simulink model "BasePendulumSim"  (R2018b)
settings: Solver=VariableStepAuto  StartTime=0.0  StopTime=time(end)  RelTol=1e-3
values from neighbouring files (symbols this model uses):
  B = 0.25    [BasePendulumTest.m]
  g = 9.81    [BasePendulumTest.m]    (also in FeedbackSimOptimization.m; FeedbackSimTest.m; SimVariables.mat)
  ICs = [pi 0]    [BasePendulumTest.m]    (also in FeedbackSimOptimization.m; FeedbackSimTest.m = [pi/2 0]; SimVariables.mat = [3.14159265359 0])
  K = 1    [BasePendulumTest.m]
  L = 0.2    [BasePendulumTest.m]    (also in FeedbackSimOptimization.m; FeedbackSimTest.m; SimVariables.mat)
  m = 4    [BasePendulumTest.m]    (also in FeedbackSimOptimization.m; FeedbackSimTest.m; SimVariables.mat)
  PertAmplitude = -1*[0 1 2 5]    [BasePendulumTest.m]    (also in FeedbackSimOptimization.m = -1; FeedbackSimTest.m = 0; SimVariables.mat = -1)
  PertDelay = 1    [BasePendulumTest.m]    (also in FeedbackSimOptimization.m = 0.1; FeedbackSimTest.m = 3; SimVariables.mat = 0.1)
  PertPeriod = time(end)    [BasePendulumTest.m]    (also in FeedbackSimOptimization.m; FeedbackSimTest.m; SimVariables.mat = 0.6)
  PertWidth = 5    [BasePendulumTest.m]    (also in FeedbackSimOptimization.m = 10; FeedbackSimTest.m = 10; SimVariables.mat = 10)
  Theta0 = pi    (= 3.14159265359)    [BasePendulumTest.m]
settings Model: Creator=seboe  LastModifiedBy=seboe

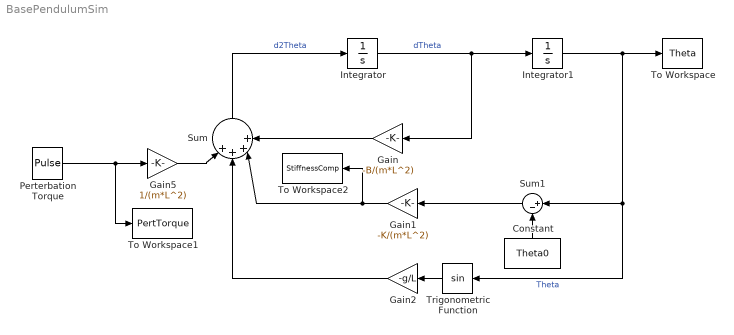
== system BasePendulumSim ==
  Constant : Constant  Value=Theta0
  Gain : Gain  Gain=-B/(m*L^2)
  Gain1 : Gain  Gain=-K/(m*L^2)
  Gain2 : Gain  Gain=-g/L
  Gain5 : Gain  Gain=1/(m*L^2)
  Integrator : Integrator  InitialCondition=ICs(2)
  Integrator1 : Integrator  InitialCondition=ICs(1)
  Perterbation Torque : DiscretePulseGenerator  PulseType=Time based  Amplitude=PertAmplitude  Period=PertPeriod  PulseWidth=PertWidth  PhaseDelay=PertDelay
  Sum : Sum  Inputs=|++++
  Sum1 : Sum  Inputs=|+-
  To Workspace : ToWorkspace  VariableName=Theta  SaveFormat=Timeseries  SampleTime=-1
  To Workspace1 : ToWorkspace  VariableName=PertTorque  SaveFormat=Timeseries  SampleTime=-1
  To Workspace2 : ToWorkspace  VariableName=StiffnessComp  SaveFormat=Timeseries  SampleTime=-1
  Trigonometric Function : Trigonometry
  wires:
  Integrator1/1 -> Sum1/1, Trigonometric Function/1, To Workspace/1  "Theta"
  Gain2/1 -> Sum/2
  Gain1/1 -> To Workspace2/1, Sum/3
  Gain/1 -> Sum/4
  Sum/1 -> Integrator/1  "d2Theta"
  Integrator/1 -> Gain/1, Integrator1/1  "dTheta"
  Gain5/1 -> Sum/1
  Perterbation Torque/1 -> Gain5/1, To Workspace1/1
  Trigonometric Function/1 -> Gain2/1
  Sum1/1 -> Gain1/1
  Constant/1 -> Sum1/2
